simulink library "gps_block"  (R2025b)
settings: Solver=VariableStepAuto  StartTime=0.0  StopTime=10.0  RelTol=1e-3
values from neighbouring files (symbols this model uses):
  GPS = evalin('base', 'GPS')    [test_gps_model.m]
settings Model: Creator=Ashwin  LastModifiedBy=Ashwin

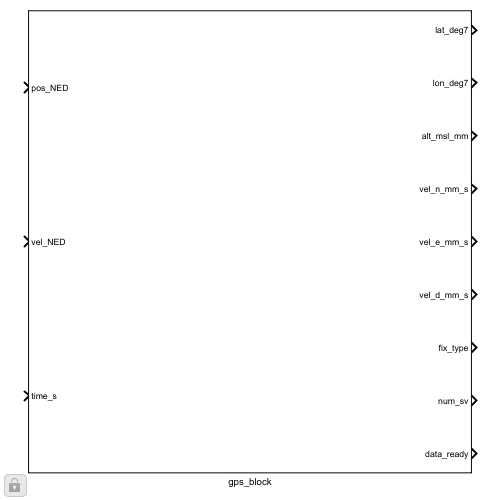
[thumbnail: Simulink's stored preview of the top-level diagram]
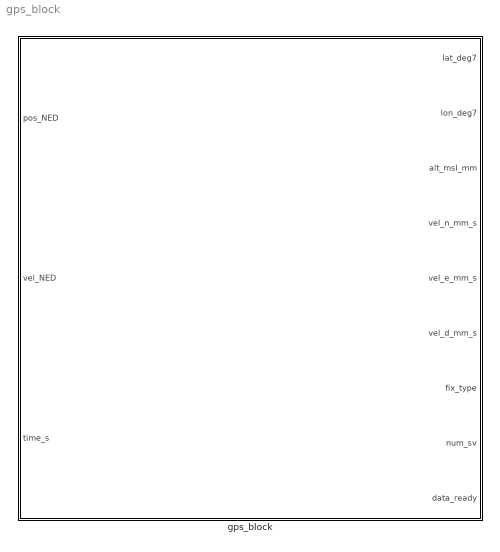
== system gps_block ==
  gps_block : Subsystem

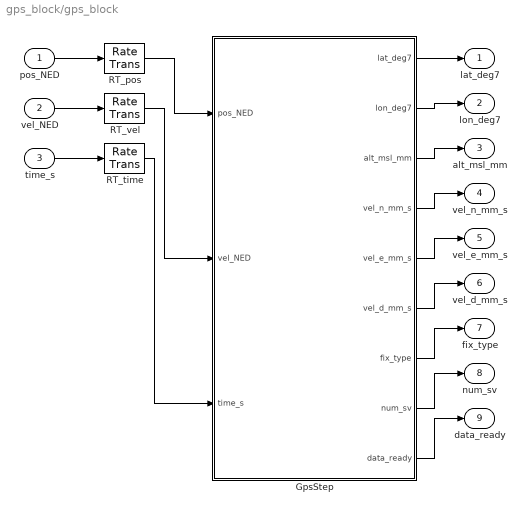
== system gps_block/gps_block ==
  pos_NED : Inport  PortDimensions=3
  vel_NED : Inport  Port=2  PortDimensions=3
  time_s : Inport  Port=3  PortDimensions=1
  GpsStep : MATLAB Function  TreatAsAtomicUnit=on
  RT_pos : RateTransition  OutPortSampleTime=1/GPS.Rate_Hz
  RT_time : RateTransition  OutPortSampleTime=1/GPS.Rate_Hz
  RT_vel : RateTransition  OutPortSampleTime=1/GPS.Rate_Hz
  lat_deg7 : Outport  PortDimensions=1
  lon_deg7 : Outport  Port=2  PortDimensions=1
  alt_msl_mm : Outport  Port=3  PortDimensions=1
  vel_n_mm_s : Outport  Port=4  PortDimensions=1
  vel_e_mm_s : Outport  Port=5  PortDimensions=1
  vel_d_mm_s : Outport  Port=6  PortDimensions=1
  fix_type : Outport  Port=7  PortDimensions=1
  num_sv : Outport  Port=8  PortDimensions=1
  data_ready : Outport  Port=9  PortDimensions=1
  wires:
  pos_NED/1 -> RT_pos/1
  vel_NED/1 -> RT_vel/1
  time_s/1 -> RT_time/1
  RT_pos/1 -> GpsStep/1(pos_NED)
  RT_vel/1 -> GpsStep/2(vel_NED)
  RT_time/1 -> GpsStep/3(time_s)
  GpsStep/1(lat_deg7) -> lat_deg7/1
  GpsStep/2(lon_deg7) -> lon_deg7/1
  GpsStep/3(alt_msl_mm) -> alt_msl_mm/1
  GpsStep/4(vel_n_mm_s) -> vel_n_mm_s/1
  GpsStep/5(vel_e_mm_s) -> vel_e_mm_s/1
  GpsStep/6(vel_d_mm_s) -> vel_d_mm_s/1
  GpsStep/7(fix_type) -> fix_type/1
  GpsStep/8(num_sv) -> num_sv/1
  GpsStep/9(data_ready) -> data_ready/1

== matlab function gps_block/GpsStep ==
  data: pos_NED input; lat_deg7 output; vel_NED input; time_s input; lon_deg7 output; alt_msl_mm output; vel_n_mm_s output; vel_e_mm_s output; vel_d_mm_s output; fix_type output; num_sv output; data_ready output
function [lat_deg7, lon_deg7, alt_msl_mm, ...
          vel_n_mm_s, vel_e_mm_s, vel_d_mm_s, ...
          fix_type, num_sv, data_ready] = GpsStep(pos_NED, vel_NED, time_s)
%#codegen
coder.extrinsic('evalin');
coder.extrinsic('casper_gps_step');

% Default-initialise outputs so the codegen-time types are known.
lat_deg7    = int32(0);
lon_deg7    = int32(0);
alt_msl_mm  = int32(0);
vel_n_mm_s  = int32(0);
vel_e_mm_s  = int32(0);
vel_d_mm_s  = int32(0);
fix_type    = uint8(0);
num_sv      = uint8(0);
data_ready  = false;

% Pull parameters from the base workspace at run time. Defaults are
% only used at codegen for type inference; the evalin calls overwrite
% them every simulation step.
lat0_deg       = 0.0;
lon0_deg       = 0.0;
alt0_m         = 0.0;
earth_radius_m = 6371000.0;
sigma_h_m      = 0.0;
sigma_v_m      = 0.0;
sigma_vel_mps  = 0.0;
vel_thresh_mps = 500.0;
alt_thresh_m   = 18000.0;
reacquire_s    = 1.0;
seed           = uint32(0);

lat0_deg       = evalin('base', 'GPS_local.LaunchLat_deg');
lon0_deg       = evalin('base', 'GPS_local.LaunchLon_deg');
alt0_m         = evalin('base', 'GPS_local.LaunchAlt_m');
earth_radius_m = evalin('base', 'GPS_local.EarthRadius_m');
sigma_h_m      = evalin('base', 'GPS_local.PositionSigmaHorizontal_m');
sigma_v_m      = evalin('base', 'GPS_local.PositionSigmaVertical_m');
sigma_vel_mps  = evalin('base', 'GPS_local.VelocitySigma_mps');
vel_thresh_mps = evalin('base', 'GPS_local.COCOMVelThreshold_mps');
alt_thresh_m   = evalin('base', 'GPS_local.COCOMAltThreshold_m');
reacquire_s    = evalin('base', 'GPS_local.ReacquireTime_s');
seed           = uint32(evalin('base', 'GPS_local.Seed'));

[lat_deg7, lon_deg7, alt_msl_mm, ...
 vel_n_mm_s, vel_e_mm_s, vel_d_mm_s, ...
 fix_type, num_sv, data_ready] = casper_gps_step( ...
    pos_NED, vel_NED, time_s, ...
    lat0_deg, lon0_deg, alt0_m, earth_radius_m, ...
    sigma_h_m, sigma_v_m, sigma_vel_mps, ...
    vel_thresh_mps, alt_thresh_m, reacquire_s, seed);
end
